simulink model "RESE412_A2_Simulink"  (R2025b)
settings: Solver=VariableStepAuto  StartTime=0.0  StopTime=5  RelTol=1e-3
values from neighbouring files (symbols this model uses):
  c0_12 = kc*c1_12    (= 5.4e-09)    [RESE412_A2.m]
  c0_23 = kc*c1_23    (= 5.4e-09)    [RESE412_A2.m]
  c0_25 = kc*c1_25    (= 5.1e-09)    [RESE412_A2.m]
  c1_12 = 9e-9    (= 9e-09)    [RESE412_A2.m]
  c1_23 = 9e-9    (= 9e-09)    [RESE412_A2.m]
  c1_25 = 8.5e-9    (= 8.5e-09)    [RESE412_A2.m]
  f = 50    [RESE412_A2.m]
  f_tr = 50    [RESE412_A2.m]
  l0_12 = kl*l1_12    (= 0.003465)    [RESE412_A2.m]
  l0_23 = kl*l1_23    (= 0.003465)    [RESE412_A2.m]
  l0_25 = kl*l1_25    (= 0.003135)    [RESE412_A2.m]
  l1_12 = 1.05e-3    (= 0.00105)    [RESE412_A2.m]
  l1_23 = 1.05e-3    (= 0.00105)    [RESE412_A2.m]
  l1_25 = 0.95e-3    (= 0.00095)    [RESE412_A2.m]
  L_g = X_g / (2*pi*f)    [RESE412_A2.m]
  L_tr_1 = L_tr_total/2    (= 0.04)    [RESE412_A2.m]
  L_tr_2 = L_tr_total/2    (= 0.04)    [RESE412_A2.m]
  r0_12 = kr*r1_12    (= 0.368)    [RESE412_A2.m]
  r0_23 = kr*r1_23    (= 0.368)    [RESE412_A2.m]
  r0_25 = kr*r1_25    (= 0.576)    [RESE412_A2.m]
  r1_12 = 0.115    [RESE412_A2.m]
  r1_23 = 0.115    [RESE412_A2.m]
  r1_25 = 0.180    (= 0.18)    [RESE412_A2.m]
  R_g = X_g / XR    [RESE412_A2.m]
  R_tr_1 = R_tr_total/2    (= 0.002)    [RESE412_A2.m]
  R_tr_2 = R_tr_total/2    (= 0.002)    [RESE412_A2.m]
  S_tr = 1.5e6    (= 1500000)    [RESE412_A2.m]
  t_switch = 2    [RESE412_A2.m]
  V_grid = 110e3    (= 110000)    [RESE412_A2.m]
  V_HV = 110e3    (= 110000)    [RESE412_A2.m]
  V_LV = 11e3    (= 11000)    [RESE412_A2.m]
undefined symbols (not defined in the file or in its folder): D11, Delta
libraries: spsThreePhaseVIMeasurementLib x5, spsThreePhasePISectionLineLib x4, spsBreakerLib x3, spsThreePhaseSeriesRLCLoadLib x2, Helpful_Lib_2 x1, spsRMSLib x1, dspstat3 x1, spsThreePhaseTransformerTwoWindingsLib x1, spsThreePhaseSourceLib x1, sps_lib x1, spspowerguiLib x1
settings Model: Creator=Cullum  LastModifiedBy=toumoucull

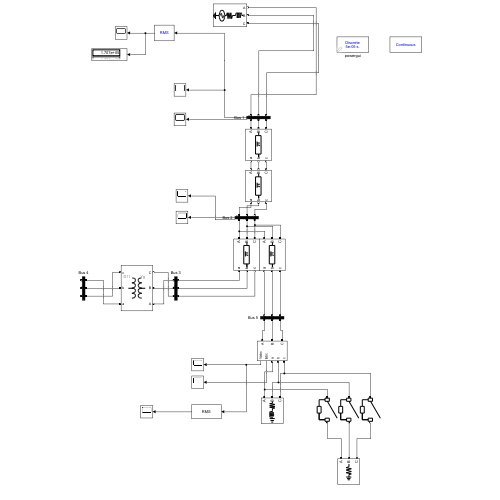
[thumbnail: Simulink's stored preview of the top-level diagram]
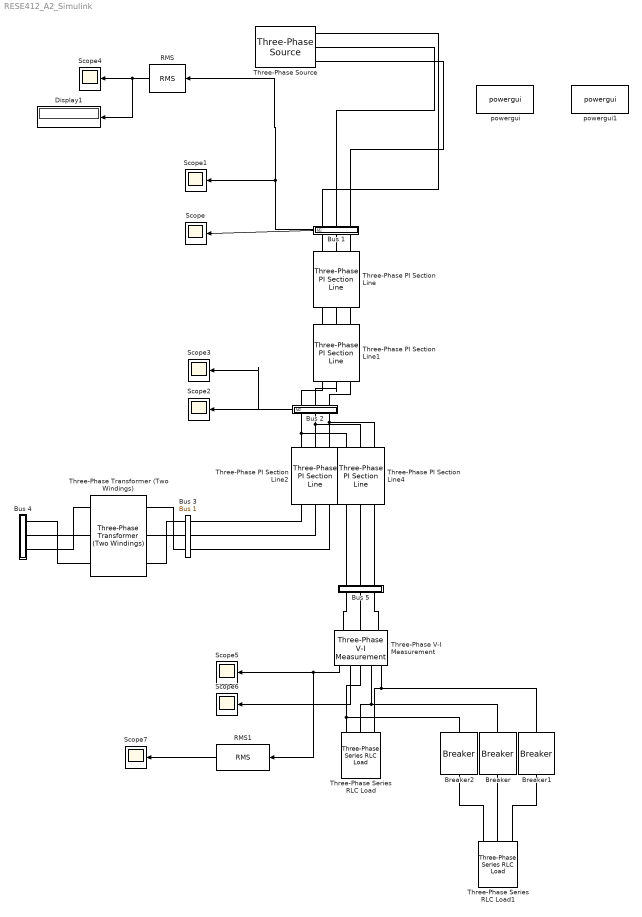
== system RESE412_A2_Simulink ==
  Breaker : spsBreakerLib/Breaker  InitialState=0  SwitchingTimes=[t_switch]  External=off  BreakerResistance=0.01  SnubberResistance=1e6  SnubberCapacitance=inf  Measurements=None  MoreParameters=on  NoBreakLoop=off
  Breaker1 : spsBreakerLib/Breaker  InitialState=0  SwitchingTimes=[t_switch]  External=off  BreakerResistance=0.01  SnubberResistance=1e6  SnubberCapacitance=inf  Measurements=None  MoreParameters=on  NoBreakLoop=off
  Breaker2 : spsBreakerLib/Breaker  InitialState=0  SwitchingTimes=[t_switch]  External=off  BreakerResistance=0.01  SnubberResistance=1e6  SnubberCapacitance=inf  Measurements=None  MoreParameters=on  NoBreakLoop=off
  Bus 1 : Subsystem  AncestorBlock=Helpful_Lib_2/Bus 1
      settings: PortSchema="{\"entries\":[{\"content\":{\"sides\":[{\"content\":{},\"type\":\"ConnectorPlacement.EquallySpacedRectSide\",\"uuid\":\"be7d712d-2536-4b6d-807b-febc1b7dbc84\"},{\"content\":{\"connectorIds\":[\"Out1\",\"Out2\"],\"side\":\"RIGHT\"},\"type\":\"ConnectorPlacement.EquallySpacedRectSide\",\"uuid\":\"94605130-94af-4a6c-ba2a-ab564513d197\"},{\"content\":{\"connectorIds\":[\"LConn1\",\"LConn2\",\"LConn3\"],\"side\":\"TOP\"},\"type\":\"ConnectorPlacement.EquallySpacedRectSide\",\"uuid\":\"3248bbab-3c18-44e8-a8cc-b027e3a839ec\"},{\"content\":{\"connectorIds\":[\"RConn1\",\"RConn2\",\"RConn3\"],\"side\":\"BOTTOM\"},\"type\":\"ConnectorPlacement.EquallySpacedRectSide\",\"uuid\":\"8fcae213-7121-4d6d-9f96-df757f1a6414\"}]},\"type\":\"ConnectorPlacement.EquallySpacedConnector\",\"uuid\":\"e1a58a3c-7f8e-4395-9b7a-281719746d6f\"}],\"packageUris\":[\"http://schema.mathworks.com/mf0/Connector/R2020b\"],\"version\":\"1.0\"}"
  Bus 2 : Subsystem  AncestorBlock=Helpful_Lib_2/Bus 1
      settings: PortSchema="{\"entries\":[{\"content\":{\"sides\":[{\"content\":{},\"type\":\"ConnectorPlacement.EquallySpacedRectSide\",\"uuid\":\"be7d712d-2536-4b6d-807b-febc1b7dbc84\"},{\"content\":{\"connectorIds\":[\"Out1\",\"Out2\"],\"side\":\"RIGHT\"},\"type\":\"ConnectorPlacement.EquallySpacedRectSide\",\"uuid\":\"94605130-94af-4a6c-ba2a-ab564513d197\"},{\"content\":{\"connectorIds\":[\"LConn1\",\"LConn2\",\"LConn3\"],\"side\":\"TOP\"},\"type\":\"ConnectorPlacement.EquallySpacedRectSide\",\"uuid\":\"3248bbab-3c18-44e8-a8cc-b027e3a839ec\"},{\"content\":{\"connectorIds\":[\"RConn1\",\"RConn2\",\"RConn3\"],\"side\":\"BOTTOM\"},\"type\":\"ConnectorPlacement.EquallySpacedRectSide\",\"uuid\":\"8fcae213-7121-4d6d-9f96-df757f1a6414\"}]},\"type\":\"ConnectorPlacement.EquallySpacedConnector\",\"uuid\":\"e1a58a3c-7f8e-4395-9b7a-281719746d6f\"}],\"packageUris\":[\"http://schema.mathworks.com/mf0/Connector/R2020b\"],\"version\":\"1.0\"}"
  Bus 3 : Helpful_Lib_2/Bus 1  SystemSampleTime=-1  VariantActivationTime=update diagram  EmptyChoice=off  PassThrough=off  PassThroughVariantControl=(default)  EmptyChoiceVariantControl=(default)  AllowFlexibleInterface=on  Latency=0  AutoFrameSizeCalculation=off
      settings: PortSchema="{\"entries\":[{\"content\":{\"sides\":[{\"content\":{},\"type\":\"ConnectorPlacement.EquallySpacedRectSide\",\"uuid\":\"be7d712d-2536-4b6d-807b-febc1b7dbc84\"},{\"content\":{\"side\":\"RIGHT\"},\"type\":\"ConnectorPlacement.EquallySpacedRectSide\",\"uuid\":\"94605130-94af-4a6c-ba2a-ab564513d197\"},{\"content\":{\"connectorIds\":[\"LConn1\",\"LConn2\",\"LConn3\"],\"side\":\"TOP\"},\"type\":\"ConnectorPlacement.EquallySpacedRectSide\",\"uuid\":\"3248bbab-3c18-44e8-a8cc-b027e3a839ec\"},{\"content\":{\"connectorIds\":[\"RConn1\",\"RConn2\",\"RConn3\"],\"side\":\"BOTTOM\"},\"type\":\"ConnectorPlacement.EquallySpacedRectSide\",\"uuid\":\"8fcae213-7121-4d6d-9f96-df757f1a6414\"}]},\"type\":\"ConnectorPlacement.EquallySpacedConnector\",\"uuid\":\"e1a58a3c-7f8e-4395-9b7a-281719746d6f\"}],\"packageUris\":[\"http://schema.mathworks.com/mf0/Connector/R2020b\"],\"version\":\"1.0\"}"
  Bus 4 : Subsystem  AncestorBlock=Helpful_Lib_2/Bus 1
      settings: PortSchema="{\"entries\":[{\"content\":{\"sides\":[{\"content\":{},\"type\":\"ConnectorPlacement.EquallySpacedRectSide\",\"uuid\":\"be7d712d-2536-4b6d-807b-febc1b7dbc84\"},{\"content\":{\"side\":\"RIGHT\"},\"type\":\"ConnectorPlacement.EquallySpacedRectSide\",\"uuid\":\"94605130-94af-4a6c-ba2a-ab564513d197\"},{\"content\":{\"connectorIds\":[\"LConn1\",\"LConn2\",\"LConn3\"],\"side\":\"TOP\"},\"type\":\"ConnectorPlacement.EquallySpacedRectSide\",\"uuid\":\"3248bbab-3c18-44e8-a8cc-b027e3a839ec\"},{\"content\":{\"connectorIds\":[\"RConn1\",\"RConn2\",\"RConn3\"],\"side\":\"BOTTOM\"},\"type\":\"ConnectorPlacement.EquallySpacedRectSide\",\"uuid\":\"8fcae213-7121-4d6d-9f96-df757f1a6414\"}]},\"type\":\"ConnectorPlacement.EquallySpacedConnector\",\"uuid\":\"e1a58a3c-7f8e-4395-9b7a-281719746d6f\"}],\"packageUris\":[\"http://schema.mathworks.com/mf0/Connector/R2020b\"],\"version\":\"1.0\"}"
  Bus 5 : Subsystem  AncestorBlock=Helpful_Lib_2/Bus 1
      settings: PortSchema="{\"entries\":[{\"content\":{\"sides\":[{\"content\":{},\"type\":\"ConnectorPlacement.EquallySpacedRectSide\",\"uuid\":\"be7d712d-2536-4b6d-807b-febc1b7dbc84\"},{\"content\":{\"side\":\"RIGHT\"},\"type\":\"ConnectorPlacement.EquallySpacedRectSide\",\"uuid\":\"94605130-94af-4a6c-ba2a-ab564513d197\"},{\"content\":{\"connectorIds\":[\"LConn1\",\"LConn2\",\"LConn3\"],\"side\":\"TOP\"},\"type\":\"ConnectorPlacement.EquallySpacedRectSide\",\"uuid\":\"3248bbab-3c18-44e8-a8cc-b027e3a839ec\"},{\"content\":{\"connectorIds\":[\"RConn1\",\"RConn2\",\"RConn3\"],\"side\":\"BOTTOM\"},\"type\":\"ConnectorPlacement.EquallySpacedRectSide\",\"uuid\":\"8fcae213-7121-4d6d-9f96-df757f1a6414\"}]},\"type\":\"ConnectorPlacement.EquallySpacedConnector\",\"uuid\":\"e1a58a3c-7f8e-4395-9b7a-281719746d6f\"}],\"packageUris\":[\"http://schema.mathworks.com/mf0/Connector/R2020b\"],\"version\":\"1.0\"}"
  Display1 : Display
  RMS : spsRMSLib/RMS  TrueRMS=on  Freq=50  RMSInit=120  Ts=0
  RMS1 : dspstat3/RMS  run=off  directionMode=Each column  dimension=1  InputProcessing=Columns as channels (frame based)  reset_popup=None
  Scope{,1..7} (8 alike) : Scope
      Scope settings: ActiveDisplayYMinimum=-1.3497403495440736  ActiveDisplayYMaximum=1.0812721504559273
      Scope1 settings: ActiveDisplayYMinimum=-290058.54095116077  ActiveDisplayYMaximum=290598.95712487155
      Scope2 settings: ActiveDisplayYMinimum=-1  ActiveDisplayYMaximum=1  DataLoggingVariableName=ScopeData4
      Scope3 settings: ActiveDisplayYMinimum=-1  ActiveDisplayYMaximum=1  DataLoggingVariableName=ScopeData8
      Scope4 settings: ActiveDisplayYMinimum=-1.7547775553236431E+6  ActiveDisplayYMaximum=535031.12454661448  DataLoggingVariableName=ScopeData2
      Scope5 settings: ActiveDisplayYMinimum=-282540.69717026403  ActiveDisplayYMaximum=282540.99317724421  DataLoggingVariableName=ScopeData7
      Scope6 settings: DataLoggingVariableName=ScopeData9
      Scope7 settings: ActiveDisplayYMinimum=164132.64494995103  ActiveDisplayYMaximum=230992.16377329256  DataLoggingVariableName=ScopeData10
  Three-Phase PI Section Line : spsThreePhasePISectionLineLib/Three-Phase PI Section Line  LConnTagsString=a|b|c  RConnTagsString=A|B|C  Length=L12_1  Frequency=f  Resistances=[r1_12 r0_12]  Inductances=[l1_12 l0_12]  Capacitances=[c1_12 c0_12]
  Three-Phase PI Section Line1 : spsThreePhasePISectionLineLib/Three-Phase PI Section Line  LConnTagsString=a|b|c  RConnTagsString=A|B|C  Length=L12_2  Frequency=f  Resistances=[r1_12 r0_12]  Inductances=[l1_12 l0_12]  Capacitances=[c1_12 c0_12]
  Three-Phase PI Section Line2 : spsThreePhasePISectionLineLib/Three-Phase PI Section Line  LConnTagsString=a|b|c  RConnTagsString=A|B|C  Length=L23  Frequency=f  Resistances=[r1_23 r0_23]  Inductances=[l1_23 l0_23]  Capacitances=[c1_23 c0_23]
  Three-Phase PI Section Line4 : spsThreePhasePISectionLineLib/Three-Phase PI Section Line  LConnTagsString=a|b|c  RConnTagsString=A|B|C  Length=L25  Frequency=f  Resistances=[r1_25 r0_25]  Inductances=[l1_25 l0_25]  Capacitances=[c1_25 c0_25]
  Three-Phase Series RLC Load : spsThreePhaseSeriesRLCLoadLib/Three-Phase Series RLC Load  LConnTagsString=A|B|C  Configuration=Y (grounded)  NominalVoltage=V_grid  Vabc=[1e3 1e3 1e3]  Vabcp=[1e3 1e3 1e3]  NominalFrequency=f  UnbalancedPower=off  ActivePower=500e3  InductivePower=150e3  CapacitivePower=0  Pabc=[10e3 9e3 11e3]  QLabc=[100 90 110]  QCabc=[100 90 110]  Pabcp=[10e3 9e3 11e3]  QLabcp=[100 90 110]  QCabcp=[100 90 110]  Measurements=None  LoadType=constant Z
  Three-Phase Series RLC Load1 : spsThreePhaseSeriesRLCLoadLib/Three-Phase Series RLC Load  LConnTagsString=A|B|C  Configuration=Y (grounded)  NominalVoltage=V_grid  Vabc=[1e3 1e3 1e3]  Vabcp=[1e3 1e3 1e3]  NominalFrequency=f  UnbalancedPower=off  ActivePower=250e3  InductivePower=0  CapacitivePower=0  Pabc=[10e3 9e3 11e3]  QLabc=[100 90 110]  QCabc=[100 90 110]  Pabcp=[10e3 9e3 11e3]  QLabcp=[100 90 110]  QCabcp=[100 90 110]  Measurements=None  LoadType=constant Z
  Three-Phase Transformer (Two Windings) : spsThreePhaseTransformerTwoWindingsLib/Three-Phase Transformer (Two Windings)  Winding1Connection=Yg  Winding2Connection=Delta (D11)  CoreType=Three single-phase transformers  SetSaturation=off  Hysteresis=off  DataFile='hysteresis'  SetInitialFlux=off  Measurements=None  UNITS=pu  NominalPower=[S_tr f_tr]  Winding1=[V_HV R_tr_1 L_tr_1]  Winding2=[V_LV R_tr_2 L_tr_2]  Rm=500  Lm=500  L0=0.5  Saturation=[ 0,0 ; 0.0024,1.2 ; 1.0,1.52 ]  InitialFluxes=[ 0.8 , -0.8 , 0.7 ]  BreakLoop=off  DiscreteSolver=Trapezoidal iterative  DataType=off  TransfoNumber=1
  Three-Phase V-I Measurement : spsThreePhaseVIMeasurementLib/Three-Phase V-I Measurement  VoltageMeasurement=phase-to-phase  SetLabelV=off  LabelV=Vabc  Vpu=off  VpuLL=off  CurrentMeasurement=yes  SetLabelI=off  LabelI=Iabc  Ipu=off  Pbase=100e6  Vbase=500e3  OutputType=Complex  PhasorSimulation=off  PSBequivalent=0
  Three-Phase Source : spsThreePhaseSourceLib/Three-Phase Source  InternalConnection=Yg  VoltagePhases=off  Voltage=V_grid  PhaseAngle=0  Voltage_phases=[25e3 25e3 25e3]/sqrt(3)  PhaseAngles_phases=[0 -120 +120]  Frequency=f  NonIdealSource=on  SpecifyImpedance=off  Resistance=R_g  Inductance=L_g  ShortCircuitLevel=100e6  BaseVoltage=V_grid  XRratio=7  BusType=swing  Pref=10e3  Qref=0  Prefabc=[10e3, 10e3, 10e3]  Qrefabc=[0, 0, 0]  Qmin=-inf  Qmax=inf
  powergui : sps_lib/powergui  Priority=1  SimulationMode=Discrete  SampleTime=50e-6  frequency=60  Iterations=50  frequencyindice=50  Pbase=100e6  ErrMax=1e-4  UnitsV=kV  UnitsW=MW  buscounter=0  FunctionMessages=off  echomessages=off  EnableUseOfTLC=off  CurrentSourceSwitches=off  DisableSnubberDevices=off  DisableRonSwitches=off  DisableVfSwitches=off  DisplayEquations=off  AutomaticDiscreteSolvers=off  SolverType=Tustin/Backward Euler (TBE)  Interpol=off  ExternalGateDelay=off  methode=off  Ts=100  x0status=blocks  SPID=on  SwTol=0  HookPort=off  NonlinearTolerance=1e-4  nMaxIteration=100  ContinueOnMaxIteration=off  RestoreLinks=warning  ResistiveCurrentMeasurement=off  Frange=[0:2:500]  Ylog=off  Xlog=on  ShowGrid=off  save=off  variable=ZData  structure=0  ZoomFFT=off  StartTime=0.0  cycles=1  DisplayStyle=1  fundamental=60  FreqAxis=off  MaxFrequency=1000  frequencyindicesteady=1  RmsSteady=1  display=off
  powergui1 : spspowerguiLib/powergui  Priority=1  SimulationMode=Continuous  SampleTime=50e-6  frequency=60  Iterations=50  frequencyindice=60  Pbase=100e6  ErrMax=1e-4  UnitsV=kV  UnitsW=MW  buscounter=0  FunctionMessages=off  echomessages=off  EnableUseOfTLC=off  CurrentSourceSwitches=off  DisableSnubberDevices=off  DisableRonSwitches=off  DisableVfSwitches=off  DisplayEquations=off  AutomaticDiscreteSolvers=off  SolverType=Tustin/Backward Euler (TBE)  Interpol=off  ExternalGateDelay=off  methode=off  Ts=100  x0status=blocks  SPID=on  SwTol=0  HookPort=off  NonlinearTolerance=1e-4  nMaxIteration=100  ContinueOnMaxIteration=off  RestoreLinks=warning  ResistiveCurrentMeasurement=off  Frange=[0:2:500]  Ylog=off  Xlog=on  ShowGrid=off  save=off  variable=ZData  structure=0  ZoomFFT=off  StartTime=0.0  cycles=1  DisplayStyle=1  fundamental=60  FreqAxis=off  MaxFrequency=1000  frequencyindicesteady=1  RmsSteady=1  display=off
  wires:
  Bus 1/2(I1) -> Scope/1
  Bus 1/1(V1) -> RMS/1, Scope1/1
  Bus 2/1(I2) -> Scope2/1
  Bus 2/2(V2) -> Scope3/1
  RMS/1 -> Display1/1, Scope4/1
  Three-Phase V-I Measurement/1 -> RMS1/1, Scope5/1
  Three-Phase V-I Measurement/2 -> Scope6/1
  RMS1/1 -> Scope7/1
  connections:
  Bus 1/RConn3 -- Three-Phase PI Section Line/LConn1
  Bus 1/RConn2 -- Three-Phase PI Section Line/LConn2
  Bus 1/RConn1 -- Three-Phase PI Section Line/LConn3
  Three-Phase PI Section Line/RConn1 -- Three-Phase PI Section Line1/LConn1
  Three-Phase PI Section Line/RConn2 -- Three-Phase PI Section Line1/LConn2
  Three-Phase PI Section Line/RConn3 -- Three-Phase PI Section Line1/LConn3
  Bus 2/RConn3 -- Three-Phase PI Section Line4/LConn1 -- Three-Phase PI Section Line2/LConn1
  Bus 2/RConn2 -- Three-Phase PI Section Line4/LConn2 -- Three-Phase PI Section Line2/LConn2
  Bus 2/RConn1 -- Three-Phase PI Section Line4/LConn3 -- Three-Phase PI Section Line2/LConn3
  Three-Phase PI Section Line2/RConn1 -- Bus 3/LConn3
  Three-Phase PI Section Line2/RConn2 -- Bus 3/LConn2
  Three-Phase PI Section Line2/RConn3 -- Bus 3/LConn1
  Bus 5/LConn3 -- Three-Phase PI Section Line4/RConn1
  Bus 5/LConn2 -- Three-Phase PI Section Line4/RConn2
  Bus 5/LConn1 -- Three-Phase PI Section Line4/RConn3
  Breaker2/LConn1 -- Three-Phase Series RLC Load/LConn1 -- Three-Phase V-I Measurement/RConn1
  Breaker/LConn1 -- Three-Phase Series RLC Load/LConn2 -- Three-Phase V-I Measurement/RConn2
  Breaker1/LConn1 -- Three-Phase Series RLC Load/LConn3 -- Three-Phase V-I Measurement/RConn3
  Three-Phase PI Section Line1/RConn2 -- Bus 2/LConn2
  Three-Phase PI Section Line1/RConn3 -- Bus 2/LConn1
  Bus 2/LConn3 -- Three-Phase PI Section Line1/RConn1
  Bus 1/LConn3 -- Three-Phase Source/RConn1
  Bus 1/LConn2 -- Three-Phase Source/RConn2
  Bus 1/LConn1 -- Three-Phase Source/RConn3
  Three-Phase Transformer (Two Windings)/RConn1 -- Bus 4/LConn3
  Three-Phase Transformer (Two Windings)/RConn2 -- Bus 4/LConn2
  Three-Phase Transformer (Two Windings)/RConn3 -- Bus 4/LConn1
  Bus 3/RConn3 -- Three-Phase Transformer (Two Windings)/LConn1
  Bus 3/RConn2 -- Three-Phase Transformer (Two Windings)/LConn2
  Bus 3/RConn1 -- Three-Phase Transformer (Two Windings)/LConn3
  Three-Phase Series RLC Load1/LConn1 -- Breaker2/RConn1
  Three-Phase Series RLC Load1/LConn2 -- Breaker/RConn1
  Three-Phase Series RLC Load1/LConn3 -- Breaker1/RConn1
  Three-Phase V-I Measurement/LConn1 -- Bus 5/RConn3
  Bus 5/RConn2 -- Three-Phase V-I Measurement/LConn2
  Three-Phase V-I Measurement/LConn3 -- Bus 5/RConn1

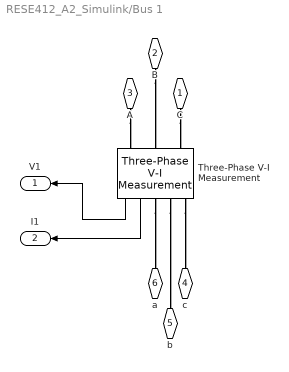
== system RESE412_A2_Simulink/Bus 1 ==
  Three-Phase V-I Measurement : spsThreePhaseVIMeasurementLib/Three-Phase V-I Measurement  VoltageMeasurement=phase-to-phase  SetLabelV=off  LabelV=Vabc  Vpu=off  VpuLL=off  CurrentMeasurement=yes  SetLabelI=off  LabelI=Iabc  Ipu=off  Pbase=100e6  Vbase=500e3  OutputType=Complex  PhasorSimulation=off  PSBequivalent=0
  C : PMIOPort  Side=Left
  B : PMIOPort  Port=2  Side=Left
  A : PMIOPort  Port=3  Side=Left
  c : PMIOPort  Port=4  Side=Right
  b : PMIOPort  Port=5  Side=Right
  a : PMIOPort  Port=6  Side=Right
  V1 : Outport
  I1 : Outport  Port=2
  wires:
  Three-Phase V-I Measurement/2 -> I1/1
  Three-Phase V-I Measurement/1 -> V1/1
  connections:
  Three-Phase V-I Measurement/RConn1 -- a/RConn1
  Three-Phase V-I Measurement/RConn2 -- b/RConn1
  A/RConn1 -- Three-Phase V-I Measurement/LConn1
  B/RConn1 -- Three-Phase V-I Measurement/LConn2
  Three-Phase V-I Measurement/RConn3 -- c/RConn1
  C/RConn1 -- Three-Phase V-I Measurement/LConn3

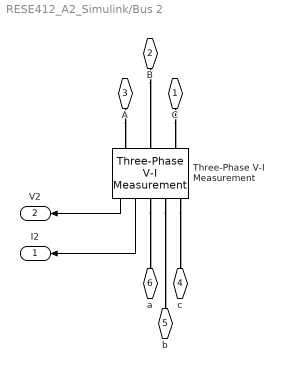
== system RESE412_A2_Simulink/Bus 2 ==
  Three-Phase V-I Measurement : spsThreePhaseVIMeasurementLib/Three-Phase V-I Measurement  VoltageMeasurement=phase-to-phase  SetLabelV=off  LabelV=Vabc  Vpu=off  VpuLL=off  CurrentMeasurement=yes  SetLabelI=off  LabelI=Iabc  Ipu=off  Pbase=100e6  Vbase=500e3  OutputType=Complex  PhasorSimulation=off  PSBequivalent=0
  C : PMIOPort  Side=Left
  B : PMIOPort  Port=2  Side=Left
  A : PMIOPort  Port=3  Side=Left
  c : PMIOPort  Port=4  Side=Right
  b : PMIOPort  Port=5  Side=Right
  a : PMIOPort  Port=6  Side=Right
  I2 : Outport
  V2 : Outport  Port=2
  wires:
  Three-Phase V-I Measurement/2 -> I2/1
  Three-Phase V-I Measurement/1 -> V2/1
  connections:
  Three-Phase V-I Measurement/RConn1 -- a/RConn1
  Three-Phase V-I Measurement/RConn2 -- b/RConn1
  A/RConn1 -- Three-Phase V-I Measurement/LConn1
  B/RConn1 -- Three-Phase V-I Measurement/LConn2
  Three-Phase V-I Measurement/RConn3 -- c/RConn1
  C/RConn1 -- Three-Phase V-I Measurement/LConn3

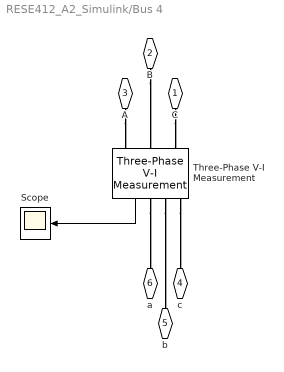
== system RESE412_A2_Simulink/Bus 4 ==
  Scope : Scope
      settings: ActiveDisplayYMinimum=-1  ActiveDisplayYMaximum=1  DataLoggingVariableName=ScopeData3
  Three-Phase V-I Measurement : spsThreePhaseVIMeasurementLib/Three-Phase V-I Measurement  VoltageMeasurement=phase-to-phase  SetLabelV=off  LabelV=Vabc  Vpu=off  VpuLL=off  CurrentMeasurement=yes  SetLabelI=off  LabelI=Iabc  Ipu=off  Pbase=100e6  Vbase=500e3  OutputType=Complex  PhasorSimulation=off  PSBequivalent=0
  C : PMIOPort  Side=Left
  B : PMIOPort  Port=2  Side=Left
  A : PMIOPort  Port=3  Side=Left
  c : PMIOPort  Port=4  Side=Right
  b : PMIOPort  Port=5  Side=Right
  a : PMIOPort  Port=6  Side=Right
  wires:
  Three-Phase V-I Measurement/2 -> Scope/1
  connections:
  Three-Phase V-I Measurement/RConn1 -- a/RConn1
  Three-Phase V-I Measurement/RConn2 -- b/RConn1
  A/RConn1 -- Three-Phase V-I Measurement/LConn1
  B/RConn1 -- Three-Phase V-I Measurement/LConn2
  Three-Phase V-I Measurement/RConn3 -- c/RConn1
  C/RConn1 -- Three-Phase V-I Measurement/LConn3

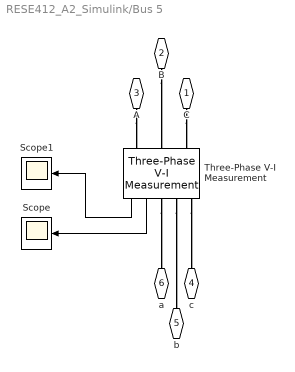
== system RESE412_A2_Simulink/Bus 5 ==
  Scope : Scope
      settings: ActiveDisplayYMinimum=0.71164599583284538  ActiveDisplayYMaximum=2.5257826515897124  DataLoggingVariableName=ScopeData5
  Scope1 : Scope
      settings: ActiveDisplayYMinimum=-548147.4922688551  ActiveDisplayYMaximum=868988.70508364507  DataLoggingVariableName=ScopeData6
  Three-Phase V-I Measurement : spsThreePhaseVIMeasurementLib/Three-Phase V-I Measurement  VoltageMeasurement=phase-to-phase  SetLabelV=off  LabelV=Vabc  Vpu=off  VpuLL=off  CurrentMeasurement=yes  SetLabelI=off  LabelI=Iabc  Ipu=off  Pbase=100e6  Vbase=500e3  OutputType=Complex  PhasorSimulation=off  PSBequivalent=0
  C : PMIOPort  Side=Left
  B : PMIOPort  Port=2  Side=Left
  A : PMIOPort  Port=3  Side=Left
  c : PMIOPort  Port=4  Side=Right
  b : PMIOPort  Port=5  Side=Right
  a : PMIOPort  Port=6  Side=Right
  wires:
  Three-Phase V-I Measurement/2 -> Scope/1
  Three-Phase V-I Measurement/1 -> Scope1/1
  connections:
  Three-Phase V-I Measurement/RConn1 -- a/RConn1
  Three-Phase V-I Measurement/RConn2 -- b/RConn1
  A/RConn1 -- Three-Phase V-I Measurement/LConn1
  B/RConn1 -- Three-Phase V-I Measurement/LConn2
  Three-Phase V-I Measurement/RConn3 -- c/RConn1
  C/RConn1 -- Three-Phase V-I Measurement/LConn3
